simulink model "Control_simu"  (R2025a)
settings: Solver=VariableStepAuto  StartTime=0.0  StopTime=25  RelTol=1e-3
values from neighbouring files (symbols this model uses):
  K = lqr(A_real,B_real,Q,R_lqr)    [Controls_proj.m]
undefined symbols (not defined in the file or in its folder): x0
settings Model: Creator=vpsom  LastModifiedBy=vpsom

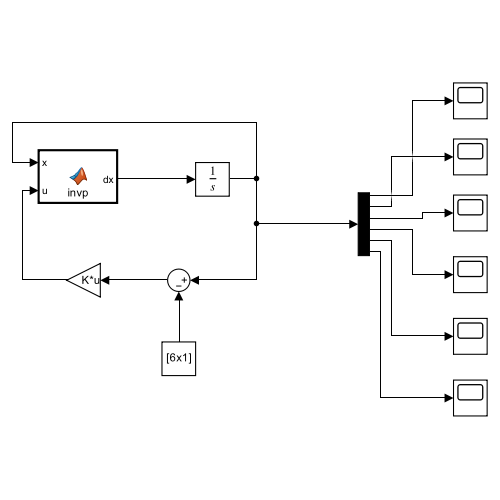
[thumbnail: Simulink's stored preview of the top-level diagram]
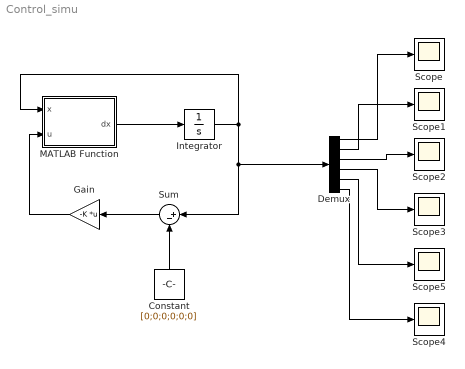
== system Control_simu ==
  Constant : Constant  Value=[0;0;0;0;0;0]
  Demux : Demux  Outputs=6
  Gain : Gain  Gain=-K  Multiplication=Matrix(K*u)
  Integrator : Integrator  InitialCondition=x0
  MATLAB Function : MATLAB Function  TreatAsAtomicUnit=on
  Scope{,1..5} (6 alike) : Scope
      Scope settings: ActiveDisplayYMinimum=-0.0037307636011333603  ActiveDisplayYMaximum=0.033576872410200249
      Scope1 settings: ActiveDisplayYMinimum=-0.024798769939145097  ActiveDisplayYMaximum=0.078043741921784829
      Scope2 settings: ActiveDisplayYMinimum=-0.019044401651217138  ActiveDisplayYMaximum=0.05767160018346857  DataLoggingVariableName=ScopeData2
      Scope3 settings: ActiveDisplayYMinimum=-0.29782597155367047  ActiveDisplayYMaximum=0.047449361590054681  DataLoggingVariableName=ScopeData3
      Scope4 settings: ActiveDisplayYMinimum=-0.02331625474498028  ActiveDisplayYMaximum=0.0451117732031662  DataLoggingVariableName=ScopeData4
      Scope5 settings: ActiveDisplayYMinimum=-0.0068679894033245488  ActiveDisplayYMaximum=0.027614734445347996  DataLoggingVariableName=ScopeData5
  Sum : Sum  Inputs=|+-
  wires:
  MATLAB Function/1(dx) -> Integrator/1
  Gain/1 -> MATLAB Function/2(u)
  Integrator/1 -> MATLAB Function/1(x), Demux/1, Sum/1
  Sum/1 -> Gain/1
  Constant/1 -> Sum/2
  Demux/1 -> Scope/1
  Demux/2 -> Scope1/1
  Demux/3 -> Scope2/1
  Demux/4 -> Scope3/1
  Demux/5 -> Scope5/1
  Demux/6 -> Scope4/1

== matlab function Control_simu/MATLAB Function ==
  data: x input; dx output; u input
function dx= invp(x, u)
    M_W = 3.4;   % kg
    R   = 0.268;  % m
    I_W = 0.5*M_W*R^2;% kg*m^2

    M_R = 12.1;   % kg
    d   = 0.21931;   % m
    h   = 0.35431;  % m
    I_yy_CoM = (1/12) * M_R * (h^2 + d^2);
    I_R = I_yy_CoM + M_R * (h/2)^2;

    m_b = 0.00274;   % kg
    r   = 0.04005;  % m
    I_b = 2/5 * m_b * r^2;

    g   = 9.81;  % m/s^2
    dx=[0;0;0;0;0;0];
    x1=x(1);
    x2=x(2);
    x3=x(3);
    x4=x(4);
    x5=x(5);
    x6=x(6);

    dx(1) = x2;
    dx(2) = -(R^3*(I_b*g*h^2*m_b^2*sin(2*x3)*abs(R)^2 - 2*I_b*R*h^2*m_b*conj(u) - 2*I_R*R*m_b*r^2*conj(u) - 2*I_b*R*m_b*r^2*conj(u) - 2*I_b*R*m_b*x5^2*conj(u) - 2*I_b*M_R*R*d^2*conj(u) - 2*R*m_b^2*r^2*x5^2*conj(u) - 2*I_R*I_b*R*conj(u) + I_R*g*m_b^2*r^2*sin(2*x3)*abs(R)^2 + I_b*g*m_b^2*r^2*sin(2*x3)*abs(R)^2 - I_b*g*m_b^2*x5^2*sin(2*x3)*abs(R)^2 - 4*I_b*R*h*m_b*r*conj(u) - 2*I_b*M_R*d*abs(R)^2*conj(u)*cos(x3) - 2*I_b*h*m_b*abs(R)^2*conj(u)*cos(x3) + 2*m_b^2*r^2*x5*abs(R)^2*conj(u)*sin(x3) - 2*I_b*m_b*r*abs(R)^2*conj(u)*cos(x3) + 2*I_b*m_b*x5*abs(R)^2*conj(u)*sin(x3) - 2*M_R*R*d^2*m_b*r^2*conj(u) + I_b*M_R^2*d^2*g*sin(2*x3)*abs(R)^2 + 2*I_b*g*h*m_b^2*x5*cos(2*x3)*abs(R)^2 + 2*I_b*g*h*m_b^2*r*sin(2*x3)*abs(R)^2 + 2*I_b*g*m_b^2*r*x5*cos(2*x3)*abs(R)^2 - 2*M_R*d*m_b*r^2*abs(R)^2*conj(u)*cos(x3) + M_R*d^2*g*m_b^2*r^2*sin(2*x3)*abs(R)^2 + M_R^2*d^2*g*m_b*r^2*sin(2*x3)*abs(R)^2 + 2*M_R*d*g*m_b^2*r^2*x5*cos(2*x3)*abs(R)^2 + 2*I_b*M_R*d*g*h*m_b*sin(2*x3)*abs(R)^2 + 2*I_b*M_R*d*g*m_b*x5*cos(2*x3)*abs(R)^2 + 2*I_b*M_R*d*g*m_b*r*sin(2*x3)*abs(R)^2))/(abs(R)^2*(2*I_R*I_b*R^3*m_b + 2*I_R*I_W*I_b*R + I_b*M_R^2*R^3*d^2 + I_b*R^3*h^2*m_b^2 + 2*I_R*I_b*M_R*R^3 + 2*I_R*I_b*M_W*R^3 + I_R*R^3*m_b^2*r^2 + I_b*R^3*m_b^2*r^2 + I_b*R^3*m_b^2*x5^2 + 2*I_b*R^3*h*m_b^2*r - I_b*M_R^2*R^3*d^2*cos(2*x3) - I_b*R^3*h^2*m_b^2*cos(2*x3) - I_R*R^3*m_b^2*r^2*cos(2*x3) - I_b*R^3*m_b^2*r^2*cos(2*x3) + I_b*R^3*m_b^2*x5^2*cos(2*x3) + 2*I_W*I_b*M_R*R*d^2 + 2*I_W*R*m_b^2*r^2*x5^2 + 2*I_W*I_b*R*h^2*m_b + 2*I_R*I_W*R*m_b*r^2 + 2*I_W*I_b*R*m_b*r^2 + 2*I_W*I_b*R*m_b*x5^2 + 2*I_b*M_R*M_W*R^3*d^2 + M_R*R^3*d^2*m_b^2*r^2 + M_R^2*R^3*d^2*m_b*r^2 + 2*M_R*R^3*m_b^2*r^2*x5^2 + 2*M_W*R^3*m_b^2*r^2*x5^2 + 2*I_b*M_R*R^3*d^2*m_b + 2*I_b*M_R*R^3*h^2*m_b + 2*I_b*M_W*R^3*h^2*m_b + 2*I_R*M_R*R^3*m_b*r^2 + 2*I_R*M_W*R^3*m_b*r^2 + 2*I_b*M_R*R^3*m_b*r^2 + 2*I_b*M_W*R^3*m_b*r^2 + 2*I_b*M_R*R^3*m_b*x5^2 + 2*I_b*M_W*R^3*m_b*x5^2 - 2*I_b*R^3*h*m_b^2*r*cos(2*x3) + 2*I_W*M_R*R*d^2*m_b*r^2 + 2*I_b*R^3*h*m_b^2*x5*sin(2*x3) + 2*I_b*R^3*m_b^2*r*x5*sin(2*x3) + 4*I_W*I_b*R*h*m_b*r + 2*M_R*M_W*R^3*d^2*m_b*r^2 - 2*I_b*M_R*R^3*d*h*m_b - 2*I_b*M_R*R^3*d*m_b*r + 4*I_b*M_R*R^3*h*m_b*r + 4*I_b*M_W*R^3*h*m_b*r - M_R*R^3*d^2*m_b^2*r^2*cos(2*x3) - M_R^2*R^3*d^2*m_b*r^2*cos(2*x3) - 2*I_b*M_R*R^3*d*h*m_b*cos(2*x3) + 2*M_R*R^3*d*m_b^2*r^2*x5*sin(2*x3) - 2*I_b*M_R*R^3*d*m_b*r*cos(2*x3) + 2*I_b*M_R*R^3*d*m_b*x5*sin(2*x3)));
    dx(3) = x4;
    dx(4) = (R*(I_b*R^3*m_b*x5*conj(u)*sin(x3) - I_b*M_R*R^2*abs(R)^2*conj(u) - I_b*M_W*R^2*abs(R)^2*conj(u) - R^2*m_b^2*r^2*abs(R)^2*conj(u) - I_b*R^2*m_b*abs(R)^2*conj(u) - I_W*m_b*r^2*abs(R)^2*conj(u) - I_W*I_b*abs(R)^2*conj(u) - M_R*R^2*m_b*r^2*abs(R)^2*conj(u) - M_W*R^2*m_b*r^2*abs(R)^2*conj(u) - I_b*M_R*R^3*d*conj(u)*cos(x3) + R^2*m_b^2*r^2*abs(R)^2*conj(u)*cos(x3)^2 - I_b*R^3*h*m_b*conj(u)*cos(x3) + R^3*m_b^2*r^2*x5*conj(u)*sin(x3) - I_b*R^3*m_b*r*conj(u)*cos(x3) + I_W*I_b*M_R*d*g*abs(R)^2*sin(x3) + I_W*g*m_b^2*r^2*x5*abs(R)^2*cos(x3) + I_W*I_b*g*h*m_b*abs(R)^2*sin(x3) + I_W*I_b*g*m_b*x5*abs(R)^2*cos(x3) + I_W*I_b*g*m_b*r*abs(R)^2*sin(x3) - M_R*R^3*d*m_b*r^2*conj(u)*cos(x3) + I_b*M_R^2*R^2*d*g*abs(R)^2*sin(x3) + I_b*R^2*g*h*m_b^2*abs(R)^2*sin(x3) + I_b*R^2*g*m_b^2*x5*abs(R)^2*cos(x3) + I_b*R^2*g*m_b^2*r*abs(R)^2*sin(x3) + I_b*M_R*M_W*R^2*d*g*abs(R)^2*sin(x3) + M_R*R^2*d*g*m_b^2*r^2*abs(R)^2*sin(x3) + M_R^2*R^2*d*g*m_b*r^2*abs(R)^2*sin(x3) + M_R*R^2*g*m_b^2*r^2*x5*abs(R)^2*cos(x3) + M_W*R^2*g*m_b^2*r^2*x5*abs(R)^2*cos(x3) + I_b*M_R*R^2*d*g*m_b*abs(R)^2*sin(x3) + I_b*M_R*R^2*g*h*m_b*abs(R)^2*sin(x3) + I_b*M_W*R^2*g*h*m_b*abs(R)^2*sin(x3) + I_b*M_R*R^2*g*m_b*x5*abs(R)^2*cos(x3) + I_b*M_W*R^2*g*m_b*x5*abs(R)^2*cos(x3) + I_b*M_R*R^2*g*m_b*r*abs(R)^2*sin(x3) + I_b*M_W*R^2*g*m_b*r*abs(R)^2*sin(x3) + I_W*M_R*d*g*m_b*r^2*abs(R)^2*sin(x3) + M_R*M_W*R^2*d*g*m_b*r^2*abs(R)^2*sin(x3)))/(abs(R)^2*(I_R*I_b*R^3*m_b + I_R*I_W*I_b*R + I_b*M_R^2*R^3*d^2 + I_b*R^3*h^2*m_b^2 + I_R*I_b*M_R*R^3 + I_R*I_b*M_W*R^3 + I_R*R^3*m_b^2*r^2 + I_b*R^3*m_b^2*r^2 + 2*I_b*R^3*h*m_b^2*r - I_b*M_R^2*R^3*d^2*cos(x3)^2 - I_b*R^3*h^2*m_b^2*cos(x3)^2 - I_R*R^3*m_b^2*r^2*cos(x3)^2 - I_b*R^3*m_b^2*r^2*cos(x3)^2 + I_b*R^3*m_b^2*x5^2*cos(x3)^2 + I_W*I_b*M_R*R*d^2 + I_W*R*m_b^2*r^2*x5^2 + I_W*I_b*R*h^2*m_b + I_R*I_W*R*m_b*r^2 + I_W*I_b*R*m_b*r^2 + I_W*I_b*R*m_b*x5^2 + I_b*M_R*M_W*R^3*d^2 + M_R*R^3*d^2*m_b^2*r^2 + M_R^2*R^3*d^2*m_b*r^2 + M_R*R^3*m_b^2*r^2*x5^2 + M_W*R^3*m_b^2*r^2*x5^2 + I_b*M_R*R^3*d^2*m_b + I_b*M_R*R^3*h^2*m_b + I_b*M_W*R^3*h^2*m_b + I_R*M_R*R^3*m_b*r^2 + I_R*M_W*R^3*m_b*r^2 + I_b*M_R*R^3*m_b*r^2 + I_b*M_W*R^3*m_b*r^2 + I_b*M_R*R^3*m_b*x5^2 + I_b*M_W*R^3*m_b*x5^2 - 2*I_b*R^3*h*m_b^2*r*cos(x3)^2 + I_W*M_R*R*d^2*m_b*r^2 + I_b*R^3*h*m_b^2*x5*sin(2*x3) + I_b*R^3*m_b^2*r*x5*sin(2*x3) + 2*I_W*I_b*R*h*m_b*r + M_R*M_W*R^3*d^2*m_b*r^2 + 2*I_b*M_R*R^3*h*m_b*r + 2*I_b*M_W*R^3*h*m_b*r - M_R*R^3*d^2*m_b^2*r^2*cos(x3)^2 - M_R^2*R^3*d^2*m_b*r^2*cos(x3)^2 - 2*I_b*M_R*R^3*d*h*m_b*cos(x3)^2 + M_R*R^3*d*m_b^2*r^2*x5*sin(2*x3) - 2*I_b*M_R*R^3*d*m_b*r*cos(x3)^2 + I_b*M_R*R^3*d*m_b*x5*sin(2*x3)));
    dx(5) = x6;
    dx(6) = (R*m_b*r^2*(I_W*r*abs(R)^2*conj(u) - I_R*R^3*conj(u)*cos(x3) + I_W*h*abs(R)^2*conj(u) - R^3*m_b*x5^2*conj(u)*cos(x3) + I_R*I_W*g*abs(R)^2*sin(x3) + M_R*R^2*h*abs(R)^2*conj(u) + M_W*R^2*h*abs(R)^2*conj(u) + M_R*R^2*r*abs(R)^2*conj(u) + M_W*R^2*r*abs(R)^2*conj(u) + R^2*h*m_b*abs(R)^2*conj(u) - M_R*R^3*d^2*conj(u)*cos(x3) + R^2*m_b*r*abs(R)^2*conj(u) - R^2*h*m_b*abs(R)^2*conj(u)*cos(x3)^2 + I_R*M_R*R^2*g*abs(R)^2*sin(x3) + I_R*M_W*R^2*g*abs(R)^2*sin(x3) - R^2*m_b*r*abs(R)^2*conj(u)*cos(x3)^2 + I_W*M_R*d^2*g*abs(R)^2*sin(x3) - R^3*h*m_b*x5*conj(u)*sin(x3) - R^3*m_b*r*x5*conj(u)*sin(x3) + (R^2*m_b*x5*sin(2*x3)*abs(R)^2*conj(u))/2 + I_R*R^2*g*m_b*abs(R)^2*sin(x3) + I_W*g*m_b*x5^2*abs(R)^2*sin(x3) + M_R*R^3*d*h*conj(u)*cos(x3) + M_R^2*R^2*d^2*g*abs(R)^2*sin(x3) + M_R*R^3*d*r*conj(u)*cos(x3) - M_R*R^2*d*abs(R)^2*conj(u)*cos(x3)^2 + M_R*R^2*g*m_b*x5^2*abs(R)^2*sin(x3) + M_W*R^2*g*m_b*x5^2*abs(R)^2*sin(x3) - I_W*M_R*d*g*h*abs(R)^2*sin(x3) - I_W*M_R*d*g*r*abs(R)^2*sin(x3) - I_W*g*h*m_b*x5*abs(R)^2*cos(x3) - I_W*g*m_b*r*x5*abs(R)^2*cos(x3) + M_R*M_W*R^2*d^2*g*abs(R)^2*sin(x3) - M_R^2*R^2*d*g*h*abs(R)^2*sin(x3) + M_R*R^2*d^2*g*m_b*abs(R)^2*sin(x3) - M_R^2*R^2*d*g*r*abs(R)^2*sin(x3) - M_R*R^2*g*h*m_b*x5*abs(R)^2*cos(x3) - M_W*R^2*g*h*m_b*x5*abs(R)^2*cos(x3) - M_R*R^2*d*g*m_b*r*abs(R)^2*sin(x3) - M_R*R^2*g*m_b*r*x5*abs(R)^2*cos(x3) - M_W*R^2*g*m_b*r*x5*abs(R)^2*cos(x3) - M_R*M_W*R^2*d*g*h*abs(R)^2*sin(x3) - M_R*M_W*R^2*d*g*r*abs(R)^2*sin(x3) - M_R*R^2*d*g*h*m_b*abs(R)^2*sin(x3) + M_R*R^2*d*g*m_b*x5*abs(R)^2*cos(x3)))/(abs(R)^2*(I_R*I_b*R^3*m_b + I_R*I_W*I_b*R + I_b*M_R^2*R^3*d^2 + I_b*R^3*h^2*m_b^2 + I_R*I_b*M_R*R^3 + I_R*I_b*M_W*R^3 + I_R*R^3*m_b^2*r^2 + I_b*R^3*m_b^2*r^2 + 2*I_b*R^3*h*m_b^2*r - I_b*M_R^2*R^3*d^2*cos(x3)^2 - I_b*R^3*h^2*m_b^2*cos(x3)^2 - I_R*R^3*m_b^2*r^2*cos(x3)^2 - I_b*R^3*m_b^2*r^2*cos(x3)^2 + I_b*R^3*m_b^2*x5^2*cos(x3)^2 + I_W*I_b*M_R*R*d^2 + I_W*R*m_b^2*r^2*x5^2 + I_W*I_b*R*h^2*m_b + I_R*I_W*R*m_b*r^2 + I_W*I_b*R*m_b*r^2 + I_W*I_b*R*m_b*x5^2 + I_b*M_R*M_W*R^3*d^2 + M_R*R^3*d^2*m_b^2*r^2 + M_R^2*R^3*d^2*m_b*r^2 + M_R*R^3*m_b^2*r^2*x5^2 + M_W*R^3*m_b^2*r^2*x5^2 + I_b*M_R*R^3*d^2*m_b + I_b*M_R*R^3*h^2*m_b + I_b*M_W*R^3*h^2*m_b + I_R*M_R*R^3*m_b*r^2 + I_R*M_W*R^3*m_b*r^2 + I_b*M_R*R^3*m_b*r^2 + I_b*M_W*R^3*m_b*r^2 + I_b*M_R*R^3*m_b*x5^2 + I_b*M_W*R^3*m_b*x5^2 - 2*I_b*R^3*h*m_b^2*r*cos(x3)^2 + I_W*M_R*R*d^2*m_b*r^2 + I_b*R^3*h*m_b^2*x5*sin(2*x3) + I_b*R^3*m_b^2*r*x5*sin(2*x3) + 2*I_W*I_b*R*h*m_b*r + M_R*M_W*R^3*d^2*m_b*r^2 + 2*I_b*M_R*R^3*h*m_b*r + 2*I_b*M_W*R^3*h*m_b*r - M_R*R^3*d^2*m_b^2*r^2*cos(x3)^2 - M_R^2*R^3*d^2*m_b*r^2*cos(x3)^2 - 2*I_b*M_R*R^3*d*h*m_b*cos(x3)^2 + M_R*R^3*d*m_b^2*r^2*x5*sin(2*x3) - 2*I_b*M_R*R^3*d*m_b*r*cos(x3)^2 + I_b*M_R*R^3*d*m_b*x5*sin(2*x3)));
end
